simulink model "Basic_1"  (R2020b)
settings: Solver=VariableStepAuto  StartTime=0.0  StopTime=20.0  RelTol=1e-3
model workspace (MAT data in the model file):
  F10 = [0  0; 0.015  28.22; 0.077  26.082; 0.201  24.934; 0.31  22.806; 0.464  20.183; 0.573  17.886; 0.789  16.075; 1.068  13.946; 1.393  12.63; 1.718  11.155; 2.166  9.844; 2.677  9.515; 3.311  9.187; 3.683  8.859; 3.791  9.679; 4.101  9.679; 4.658  9.515; 5.168  9.023; 5.725  9.023; 6.112  8.531; 6.329  8.859; 6.499  7.546; 6.685  5.742; 6.778  4.921; 6.917  2.625; 7.025  1.312; 7.13  0; 7.5  0]
  iterSeed = 0
  mountMax = 0.5
libraries: simulink_extras x3, simulink x3, shared3dof x1, pid_lib x1
settings Model: PacingRate=0.100000  Creator=jdoos  LastModifiedBy=jdoos

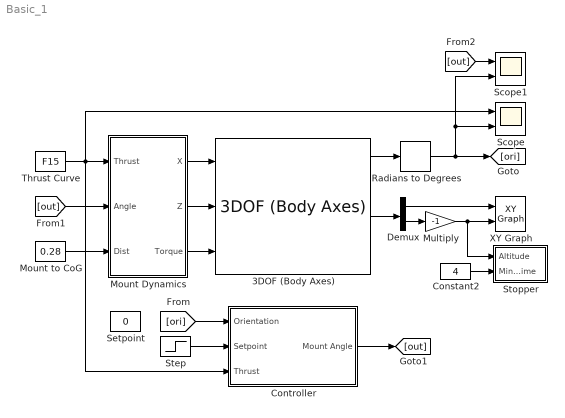
== system Basic_1 ==
  3DOF (Body Axes) : shared3dof/3DOF (Body Axes)  units=Metric (MKS)  mtype=Fixed  v_ini=0  theta_ini=0  alpha_ini=0  pos_ini=[0 0]  q_ini=0  mass=0.543  mass_e=0.5  mass_f=3.0  Iyy=0.048  Iyy_e=0.5  Iyy_f=3.0  g_in=Internal  g=9.81  vre_flag=on  abi_flag=off  aMode=0  vel_statename=''  theta_statename=''  pos_statename=''  q_statename=''  mass_statename=''
      settings: SourceProductBaseCode=AE,PW,MT,UV,VE,VP
  Constant2 : Constant  Value=4
  Controller : Subsystem
  Demux : Demux  Outputs=2
  Mount Dynamics : Subsystem
  Mount to CoG : Constant  Value=0.28
  Multiply : Gain  Gain=-1
  Radians to Degrees : simulink_extras/Transformations/Radians to Degrees
  Scope : Scope  NumInputPorts=2
  Scope1 : Scope  NumInputPorts=2
  Setpoint : Constant  Value=0
  Step : Step  Before=1  After=5  SampleTime=0
  Stopper : Subsystem
  Thrust Curve : FromWorkspace  VariableName=F15
  XY Graph : simulink/Sinks/XY Graph  xmin=-10  xmax=10  ymin=0  ymax=300  st=-1
  wires:
  Mount Dynamics/1(X) -> 3DOF (Body Axes)/1
  Mount Dynamics/2(Z) -> 3DOF (Body Axes)/2
  Mount Dynamics/3(Torque) -> 3DOF (Body Axes)/3
  Mount to CoG/1 -> Mount Dynamics/3(Dist)
  3DOF (Body Axes)/4 -> Demux/1
  Demux/1 -> XY Graph/1
  Demux/2 -> Multiply/1
  Multiply/1 -> XY Graph/2, Stopper/1(Altitude)
  Constant2/1 -> Stopper/2(Min Time)
  Thrust Curve/1 -> Controller/3(Thrust), Mount Dynamics/1(Thrust), Scope/1
  3DOF (Body Axes)/1 -> Radians to Degrees/1
  [ori] -> Controller/1(Orientation)
  Radians to Degrees/1 -> Scope/2, Scope1/2, [ori]
  [out] -> Mount Dynamics/2(Angle)
  Controller/1(Mount Angle) -> [out]
  [out] -> Scope1/1
  Step/1 -> Controller/2(Setpoint)

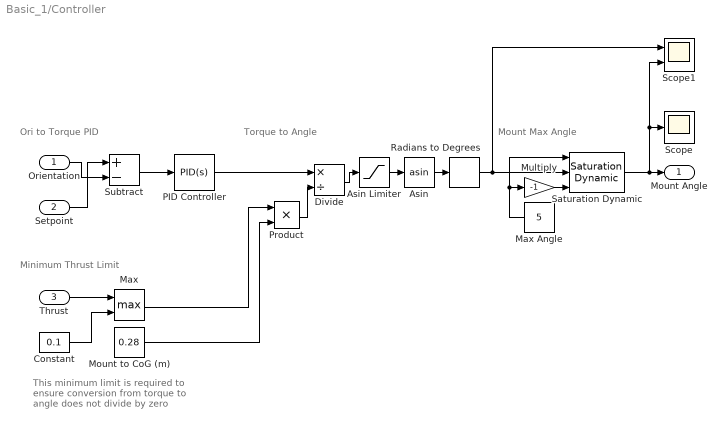
== system Basic_1/Controller ==
  note: This minimum limit is required
      | to ensure conversion from torque
      | to angle does not divide by zero
  note: Minimum Thrust Limit
  note: Mount Max Angle
  note: Torque to Angle
  note: Ori to Torque PID
  Orientation : Inport
  Setpoint : Inport  Port=2
  Thrust : Inport  Port=3
  Asin : Trigonometry  Operator=asin
  Asin Limiter : Saturate  UpperLimit=1  LowerLimit=-1
  Constant : Constant  Value=0.1
  Divide : Product  Inputs=*/
  Max : MinMax  Function=max  Inputs=2
  Max Angle : Constant  Value=5
  Mount to CoG (m) : Constant  Value=0.28
  Multiply : Gain  Gain=-1
  PID Controller : pid_lib/PID Controller  Controller=PID  Form=Ideal  TimeDomain=Continuous-time  UseExternalTs=off  SampleTime=-1  IntegratorMethod=Forward Euler  FilterMethod=Forward Euler  ControllerParametersSource=internal  P=2  I=0  D=0.2  UseFilter=on  N=100  TunerSelectOption=Transfer Function Based (PID Tuner App)  InitialConditionSource=internal  InitialConditionForIntegrator=0  InitialConditionForFilter=0  DifferentiatorICPrevScaledInput=0  ExternalReset=none  TrackingMode=off  Kt=1  LimitOutput=off  SatLimitsSource=internal  UpperSaturationLimit=inf  LowerSaturationLimit=-inf  LinearizeAsGain=on  AntiWindupMode=none  Kb=1  POutMin=[]  POutMax=[]  IOutMin=[]  IOutMax=[]  DOutMin=[]  DOutMax=[]  NOutMin=[]  NOutMax=[]  SumOutMin=[]  SumOutMax=[]  SaturationOutMin=[]  SaturationOutMax=[]  PParamMin=[]  PParamMax=[]  IParamMin=[]  IParamMax=[]  DParamMin=[]  DParamMax=[]  NParamMin=[]  NParamMax=[]  KbParamMin=[]  KbParamMax=[]  KtParamMin=[]  KtParamMax=[]  KbOutMin=[]  KbOutMax=[]  KtOutMin=[]  KtOutMax=[]  IntegratorOutMin=[]  IntegratorOutMax=[]  FilterOutMin=[]  FilterOutMax=[]  SumI1OutMin=[]  SumI1OutMax=[]  SumI2OutMin=[]  SumI2OutMax=[]  SumI3OutMin=[]  SumI3OutMax=[]  SumI4OutMin=[]  SumI4OutMax=[]  SumDOutMin=[]  SumDOutMax=[]  DifferentiatorOutMin=[]  DifferentiatorOutMax=[]  FilterDiffOutCoefMin=[]  FilterDiffOutCoefMax=[]  ReciprocalOutMin=[]  ReciprocalOutMax=[]  SumDenOutMin=[]  SumDenOutMax=[]  SumNumOutMin=[]  SumNumOutMax=[]  DivideOutMin=[]  DivideOutMax=[]  UdiffTsProdOutMin=[]  UdiffTsProdOutMax=[]  NTsProdOutMin=[]  NTsProdOutMax=[]  UintegralTsProdOutMin=[]  UintegralTsProdOutMax=[]  UngainTsProdOutMin=[]  UngainTsProdOutMax=[]  IntegratorContinuousStateAttributes=''  IntegratorStateMustResolveToSignalObject=off  IntegratorRTWStateStorageClass=Auto  FilterContinuousStateAttributes=''  FilterStateMustResolveToSignalObject=off  FilterRTWStateStorageClass=Auto  ParallelPVariant=Passthrough  IdealPVariant=InternalParameters  IVariant=InternalParameters  DVariant=InternalParameters  IntegratorVariant=Continuous  SatVariant=Disabled  AWVariant=Passthrough  PCopyVariant=Disabled  TRVariant=Disabled  FdbkBlocksVariant=Forward  IdealPFdbkVariant=Disabled  SatFdbkVariant=Disabled  DerivativeFilterVariant=ContFilter  NVariant=InternalParameters  NCopyVariant=Disabled  FilterICVariant=InternalICsFilter  IntegratorICVariant=InternalICs  ExternalResetVariant=Disabled  TRSumVariant=Passthrough  SumFdbkVariant=Disabled  SumVariant=Sum_PID  TsampFilterVariant=InternalTs  TsampNgainVariant=Passthrough  TsampIntegralVariant=Passthrough  ExternalSaturationOutDataTypeStr=Inherit: Same as second input
  Product : Product
  Radians to Degrees : simulink_extras/Transformations/Radians to Degrees
  Saturation Dynamic : simulink/Discontinuities/Saturation Dynamic  OutMin=[]  OutMax=[]  OutDataTypeStr=Inherit: Same as second input  OutDataType=fixdt(1, 16)  OutScaling=2^-10  DoSatur=off
  Scope : Scope
  Scope1 : Scope  NumInputPorts=2
  Subtract : Sum  Inputs=+-
  Mount Angle : Outport
  wires:
  Saturation Dynamic/1 -> Mount Angle/1, Scope1/2, Scope/1
  PID Controller/1 -> Divide/1
  Subtract/1 -> PID Controller/1
  Setpoint/1 -> Subtract/1
  Orientation/1 -> Subtract/2
  Multiply/1 -> Saturation Dynamic/3
  Max Angle/1 -> Saturation Dynamic/1, Multiply/1
  Product/1 -> Divide/2
  Thrust/1 -> Max/1
  Constant/1 -> Max/2
  Asin/1 -> Radians to Degrees/1
  Radians to Degrees/1 -> Scope1/1, Saturation Dynamic/2
  Asin Limiter/1 -> Asin/1
  Divide/1 -> Asin Limiter/1
  Mount to CoG (m)/1 -> Product/2
  Max/1 -> Product/1

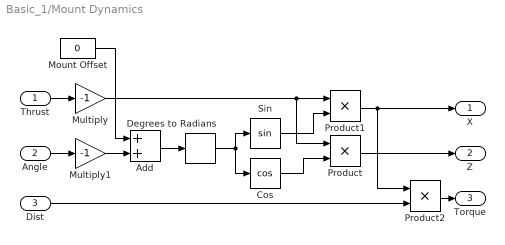
== system Basic_1/Mount Dynamics ==
  Thrust : Inport
  Angle : Inport  Port=2
  Dist : Inport  Port=3
  Add : Sum
  Cos : Trigonometry  Operator=cos
  Degrees to Radians : simulink_extras/Transformations/Degrees to Radians
  Mount Offset : Constant  Value=0
  Multiply : Gain  Gain=-1
  Multiply1 : Gain  Gain=-1
  Product : Product
  Product1 : Product
  Product2 : Product
  Sin : Trigonometry
  X : Outport
  Z : Outport  Port=2
  Torque : Outport  Port=3
  wires:
  Thrust/1 -> Multiply/1
  Sin/1 -> Product1/2
  Cos/1 -> Product/2
  Dist/1 -> Product2/2
  Product2/1 -> Torque/1
  Product1/1 -> Product2/1, X/1
  Product/1 -> Z/1
  Multiply/1 -> Product/1, Product1/1
  Angle/1 -> Multiply1/1
  Degrees to Radians/1 -> Cos/1, Sin/1
  Multiply1/1 -> Add/2
  Add/1 -> Degrees to Radians/1
  Mount Offset/1 -> Add/1

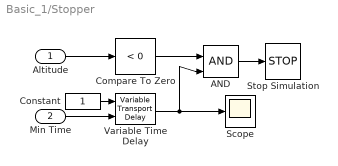
== system Basic_1/Stopper ==
  Altitude : Inport
  Min Time : Inport  Port=2
  AND : Logic  IconShape=distinctive  AllPortsSameDT=off  OutDataTypeStr=boolean
  Compare To Zero : simulink/Logic and Bit Operations/Compare To Zero  relop=<  OutDataTypeStr=boolean
  Constant : Constant
  Scope : Scope
  Stop Simulation : Stop
  Variable Time Delay : VariableTransportDelay  MaximumDelay=10
  wires:
  AND/1 -> Stop Simulation/1
  Compare To Zero/1 -> AND/1
  Altitude/1 -> Compare To Zero/1
  Variable Time Delay/1 -> Scope/1, AND/2
  Min Time/1 -> Variable Time Delay/2
  Constant/1 -> Variable Time Delay/1
